simulink model "ControladorLongitudinal"  (R2013b)
settings: Solver=ode3  StartTime=0.0  StopTime=20  FixedStep=0.002  RelTol=1e-3
values from neighbouring files (symbols this model uses):
  Alt = 1    [LoadDadosScriptSimulink.m]
  Vel = 6    [LoadDadosScriptSimulink.m]
  wa = AtSS.B(2)^0.5    [LoadDadosScriptSimulink.m]
  zetaA = -AtSS.A(2,2)/2/wa    [LoadDadosScriptSimulink.m]
undefined symbols (not defined in the file or in its folder): Kd, Kp, Plano_Long
settings Model: Creator=AGSilva  LastModifiedBy=AGSilva
settings DataIOCC: SignalLoggingSaveFormat=ModelDataLogs
settings OptimizationCC: ExpressionDepthLimit=2147483647  InitFltsAndDblsToZero=on
settings DebuggingCC: SaveWithParameterizedLinksMsg=none  FcnCallInpInsideContextMsg=UseLocalSettings  StateNameClashWarn=warning
settings SFSimCC: SimParseCustomCode=off
settings GRTTargetCC: TargetFcnLib=ansi_tfl_tmw.mat  CombineOutputUpdateFcns=off  GRTInterface=on

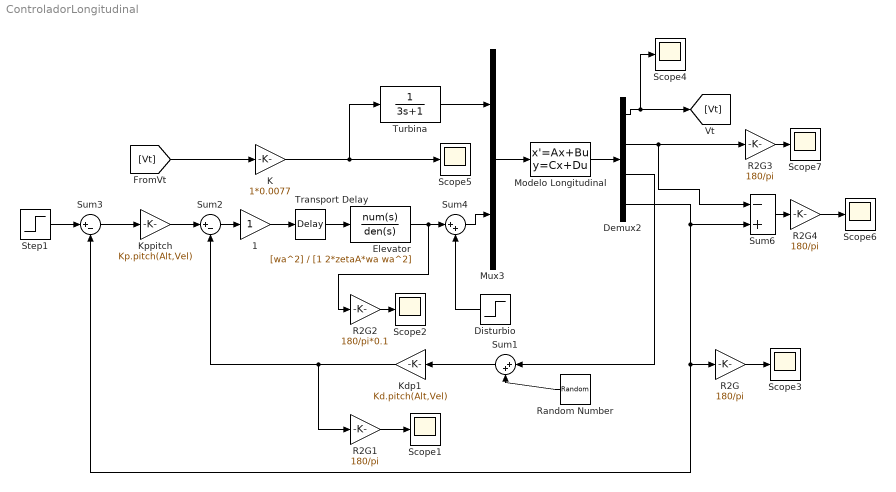
== system ControladorLongitudinal ==
  1 : Gain
  Demux2 : Demux
  Disturbio : Step  After=pi/180*0  SampleTime=0
  Elevator : TransferFcn  Numerator=[wa^2]  Denominator=[1 2*zetaA*wa wa^2]
  K : Gain  Gain=1*0.0077
  Kdp1 : Gain  Gain=Kd.pitch(Alt,Vel)
  Kppitch : Gain  Gain=Kp.pitch(Alt,Vel)
  Modelo Longitudinal : StateSpace  A=Plano_Long(Alt,Vel).A(1:4,1:4)  B=Plano_Long(Alt,Vel).B(1:4,:)  C=eye(4)  D=zeros(4,2)  X0=[0 0 0 0]'
  Mux3 : Mux  Inputs=2
  R2G{,1,3..4} (4 alike) : Gain  Gain=180/pi
  R2G2 : Gain  Gain=180/pi*0.1
  Random Number : RandomNumber  Variance=(0.002)^2*0  SampleTime=0.002
  Scope{1..7} (7 alike) : Scope
      Scope3 settings: SaveName=ScopeData3
      Scope4 settings: SaveName=ScopeData2
      Scope5 settings: SaveName=ScopeData4
      Scope6 settings: SaveName=ScopeData5
      Scope7 settings: SaveName=ScopeData6
  Step1 : Step  Time=0  After=1*pi/180  SampleTime=0
  Sum1 : Sum  Inputs=|++
  Sum2 : Sum  Inputs=|+-
  Sum3 : Sum  Inputs=|+-
  Sum4 : Sum  Inputs=|++
  Sum6 : Sum  Inputs=-+
  Transport Delay : TransportDelay  DelayTime=0.01  PadeOrder=2
  Turbina : TransferFcn  Denominator=[3 1]
  wires:
  Modelo Longitudinal/1 -> Demux2/1
  Sum3/1 -> Kppitch/1
  Kppitch/1 -> Sum2/1
  Step1/1 -> Sum3/1
  Sum1/1 -> Kdp1/1
  Random Number/1 -> Sum1/2
  Demux2/3 -> Sum1/1
  Mux3/1 -> Modelo Longitudinal/1
  Turbina/1 -> Mux3/1
  R2G/1 -> Scope3/1
  Demux2/4 -> Sum6/2, R2G/1, Sum3/2
  Demux2/2 -> Sum6/1, R2G3/1
  R2G1/1 -> Scope1/1
  Kdp1/1 -> R2G1/1, Sum2/2
  R2G2/1 -> Scope2/1
  [Vt] -> K/1
  Transport Delay/1 -> Elevator/1
  1/1 -> Transport Delay/1
  K/1 -> Turbina/1, Scope5/1
  Sum2/1 -> 1/1
  R2G4/1 -> Scope6/1
  Sum6/1 -> R2G4/1
  Demux2/1 -> Scope4/1, [Vt]
  R2G3/1 -> Scope7/1
  Elevator/1 -> R2G2/1, Sum4/1
  Sum4/1 -> Mux3/2
  Disturbio/1 -> Sum4/2
